simulink model "ModelPlant_DP_v3"  (R2014b)
settings: Solver=ode3  StartTime=0.0  StopTime=Simulation_Time  FixedStep=0.01  RelTol=1e-3
undefined symbols (not defined in the file): DesiredPath, Elipscenter_radi, eta_dot_ini, K, K1, K2, l1, l2, l3, L_1, L_2, L_3, LAW, lim, lim_2, m, mu, pd, T_initialDP, U_ref
(part 2 of 2)

== matlab function ModelPlant_DP_v3/PathParameterization/PathGenerization_Straight/Path parametization /Subsystem/MATLAB Function ==
  data: InitPosOut output; DesPos input; s_in input; U_ref input; N_iteration input; N_in input; DesPosOut output; SwitchSignal_out output; N_out output; U output; s_out output; Start_time input; init_time output; flag output
function [InitPosOut,DesPosOut,SwitchSignal_out,N_out,U,s_out,init_time,flag]= fcn(DesPos,s_in,U_ref,N_iteration,N_in,Start_time)
[a,b]=size(DesPos);
N_max=b-1;
    init_time=zeros(2,1);
    init_time(1)=Start_time(1)+1;
    init_time(2)=Start_time(2);
   
   
    
if init_time(1)<N_iteration         % DP for N_iterations
    N_out=N_in;
    InitPosOut=DesPos(:,N_out);
    DesPosOut=DesPos(:,N_out+1);
    SwitchSignal_out=1;
    s_out=0;
    DP=1;
    flag=1;
    
else
    if N_in==N_max                  % if we are at final stretch
        if  s_in>=0.9999
            N_out=N_in;
            InitPosOut=DesPos(:,N_out);
            DesPosOut=DesPos(:,N_out+1);
            SwitchSignal_out=1;
            s_out=1;
            DP=1;
            flag=2;
            
        else
            N_out=N_in;
            InitPosOut=DesPos(:,N_in);
            DesPosOut=DesPos(:,N_in+1);
            SwitchSignal_out=1;
            s_out=s_in;
            DP=0;
            flag=3;
            
        end
    else
       if s_in>=0.9999
           if N_in+1 ==N_max
               SwitchSignal_out=0;
               flag=40;
           else
               SwitchSignal_out=0;
               flag=50;
           end
            N_out=N_in+1;
            InitPosOut=DesPos(:,N_out);
            DesPosOut=DesPos(:,N_out+1);
            s_out=1;
            DP=0;

       else 
            if init_time(2)==0;
                init_time(2)=1;
                SwitchSignal_out=0;
                flag=5.75;
            else
                SwitchSignal_out=1;
                flag=5.25;
            end
            N_out=N_in;
            InitPosOut=DesPos(:,N_in);
            DesPosOut=DesPos(:,N_in+1);
            s_out=s_in;
            DP=0;
            
        end
    end
    
end   
if DP==1
    U=0;
else
    U=U_ref*(1.01+ sin(2*pi*s_out-pi/2));
end

end

== matlab function ModelPlant_DP_v3/PathParameterization/PathGenerization_Straight/parameter generator/MATLAB Function1 ==
  data: SwitchSignal_In input; SwitchSignal_Out output
function SwitchSignal_Out = fcn(SwitchSignal_In)

if SwitchSignal_In==0
    SwitchSignal_Out=1;
else
    SwitchSignal_Out=0;
end
    
end

== matlab function ModelPlant_DP_v3/PathParameterization/PathGenerization_Straight/parameter generator/UpdateLaw ==
  data: s_dot output; p_d_sdot input; U_ref input; U_s output; V_1s input; mu input; eta_ds input; LAW input
function [s_dot,U_s ]= fcn(p_d_sdot,U_ref,V_1s,mu,eta_ds,LAW)


U_s=U_ref/(sqrt(p_d_sdot(1)^2+p_d_sdot(2)^2));
if LAW ==1

        s_dot=U_s-mu*V_1s;
else
        s_dot=U_s-mu/(sqrt(eta_ds(1)^2+eta_ds(2)^2))*V_1s;
end


end

== matlab function ModelPlant_DP_v3/DPObserver1/Bias/bHatDot ==
  data: bHatDot output; L3 input; eta input; etaHat input
function bHatDot = fcn(L3,eta,etaHat)

bHatDot=L3*(eta-etaHat);
%bHatDot=[0;0;0];

end

== matlab function ModelPlant_DP_v3/DPObserver1/D ==
  data: D output; etaHatDot input
function D = fcn(etaHatDot)

u=etaHatDot(1);     %u=0; 
v=etaHatDot(2);     %v=0; 
r=etaHatDot(3);     %r=0;

Xu=-0.6555;
Xuu=0.3545;
Xuuu=-3.787;
Yv=-1.33;
Yvv=-2.776;
Yvvv=-64.91;
Yr=-7.25;
Yrr=-3.45;
Yrrr=0;
Yrv=-0.805;
Yvr=-0.845;
Nv=0;
Nvv=-0.2088;
Nvvv=0;
Nr=-1.9;
Nrr=-0.75;
Nrrr=0;
Nrv=0.13;
Nvr=0.08;

d11=-Xu-Xuu*abs(u)-Xuuu*u^2;
d22=-Yv-Yvv*abs(v)-Yvvv*v^2-Yrv*abs(r);
d23=-Yr-Yvr*abs(v)-Yrr*abs(r)-Yrrr*r^2;
d32=-Nv-Nvv*abs(v)-Nvvv*v^2-Nrv*abs(r);
d33=-Nr-Nvr*abs(v)-Nrr*abs(r)-Nrrr*r^2;

D=[d11 0 0; 0 d22 d23; 0 d32 d33];

end

== matlab function ModelPlant_DP_v3/DPObserver1/Subsystem/M ==
  data: M output
function M = void

m=14.79;
M=[m+2 0 0; 0 m+10 m*0.0375; 0 m*0.0375 1.76+1];

end

== matlab function ModelPlant_DP_v3/DPObserver1/Subsystem/nuHatDot ==
  data: nuHat input; bHat input; D input; M input; L2 input; tau input; eta input; R input; etaHat input; nuHatDot output
function nuHatDot = fcn(nuHat,bHat,D,M,L2,tau,eta,R,etaHat)

%nuHatDot=inv(M)*(-D*nuHat+transpose(R)*bHat+tau+K2*transpose(R)*L2*(eta-etaHat));

nuHatDot=inv(M)*(-D*nuHat+transpose(R)*bHat+tau+transpose(R)*L2*(eta-etaHat));

end

== matlab function ModelPlant_DP_v3/DPObserver1/calcR(psi)  ==
  data: psi input; R output
function R = fcn(psi)

R=[cos(psi) -sin(psi) 0; sin(psi) cos(psi) 0; 0 0 1];

end

== matlab function ModelPlant_DP_v3/DPObserver1/etaHat/etaHatDot ==
  data: etaHat input; nuHat input; L1 input; eta input; R input; etaHatDot output
function etaHatDot = fcn(etaHat,nuHat,L1,eta,R)

%etaHatDot=zeros(3,1);
etaHatDot=R*nuHat+L1*(eta-etaHat);

end
